simulink model "PID_temp"  (R2019b)
settings: Solver=VariableStepAuto  StartTime=0.0  StopTime=10.0  RelTol=1e-3
libraries: arduinolib x1
settings Model: Creator=sakhm  LastModifiedBy=sakhm

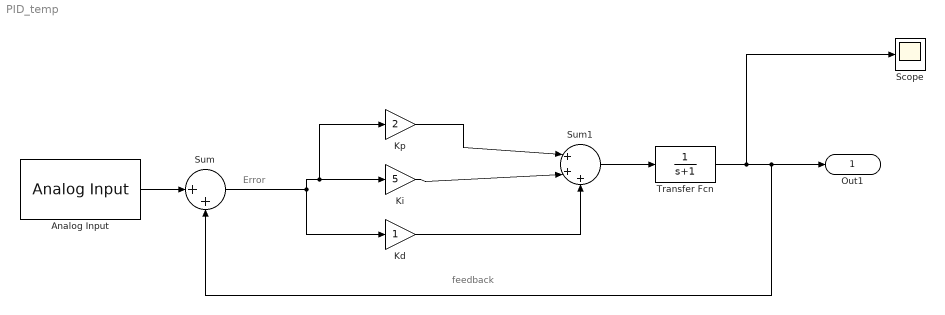
== system PID_temp ==
  note: feedback
  note: Error
  Analog Input : arduinolib/Analog Input  pinNumber=0  ReadResultsOnly=off  ConversionTriggerSource=Software  ExternalTriggerType=uint32(0)  OutputDataType=uint16  EnableConversionCompleteNotify=off  EnableOuputStatus=off  SampleTime=-1  blockPlatform=arduino
  Kd : Gain
  Ki : Gain  Gain=5
  Kp : Gain  Gain=2
  Scope : Scope
  Sum : Sum  Inputs=|++
  Sum1 : Sum  Inputs=|+++
  Transfer Fcn : TransferFcn  Denominator=[1 1]
  Out1 : Outport
  wires:
  Analog Input/1 -> Sum/1
  Sum/1 -> Ki/1, Kp/1, Kd/1
  Kp/1 -> Sum1/1
  Ki/1 -> Sum1/2
  Sum1/1 -> Transfer Fcn/1
  Transfer Fcn/1 -> Scope/1, Sum/2, Out1/1
  Kd/1 -> Sum1/3
